simulink model "control_implementation"  (R2013b)
settings: Solver=ode45  StartTime=0.0  StopTime=10.0  RelTol=1e-3
libraries: simulink x1
settings Model: Creator=tvincent  LastModifiedBy=tvincent
settings DataIOCC: SignalLoggingSaveFormat=ModelDataLogs
settings DebuggingCC: UnderspecifiedInitializationDetection=Simplified  MultiTaskDSMMsg=warning  MultiTaskCondExecSysMsg=none  StrictBusMsg=None
settings RTWCC: IncludeERTFirstTime=on
settings GRTTargetCC: CodeReplacementLibrary=None  CPPClassGenCompliant=on

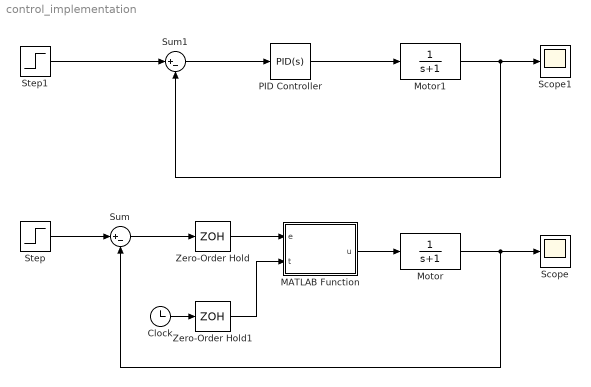
== system control_implementation ==
  Clock : Clock
  MATLAB Function : MATLAB Function  TreatAsAtomicUnit=on
  Motor : TransferFcn  Denominator=[1 1]
  Motor1 : TransferFcn  Denominator=[1 1]
  PID Controller : simulink/Continuous/PID Controller  Controller=PID  TimeDomain=Continuous-time  SampleTime=1  IntegratorMethod=Forward Euler  FilterMethod=Forward Euler  Form=Parallel  P=1  I=1  D=0  N=100  InitialConditionSource=internal  InitialConditionForIntegrator=0  InitialConditionForFilter=0  ExternalReset=none  LimitOutput=on  UpperSaturationLimit=10  LowerSaturationLimit=-10  LinearizeAsGain=on  AntiWindupMode=none  Kb=1  TrackingMode=off  Kt=1  PParamMin=[]  PParamMax=[]  IParamMin=[]  IParamMax=[]  DParamMin=[]  DParamMax=[]  NParamMin=[]  NParamMax=[]  KbParamMin=[]  KbParamMax=[]  KtParamMin=[]  KtParamMax=[]  POutMin=[]  POutMax=[]  IOutMin=[]  IOutMax=[]  DOutMin=[]  DOutMax=[]  NOutMin=[]  NOutMax=[]  KbOutMin=[]  KbOutMax=[]  KtOutMin=[]  KtOutMax=[]  IntegratorOutMin=[]  IntegratorOutMax=[]  FilterOutMin=[]  FilterOutMax=[]  SumOutMin=[]  SumOutMax=[]  SumI1OutMin=[]  SumI1OutMax=[]  SumI2OutMin=[]  SumI2OutMax=[]  SumI3OutMin=[]  SumI3OutMax=[]  SumDOutMin=[]  SumDOutMax=[]  SaturationOutMin=[]  SaturationOutMax=[]  IntegratorContinuousStateAttributes=''  IntegratorStateMustResolveToSignalObject=off  IntegratorRTWStateStorageClass=Auto  FilterContinuousStateAttributes=''  FilterStateMustResolveToSignalObject=off  FilterRTWStateStorageClass=Auto
  Scope : Scope
  Scope1 : Scope
  Step : Step  SampleTime=0
  Step1 : Step  SampleTime=0
  Sum : Sum  Inputs=|+-
  Sum1 : Sum  Inputs=|+-
  Zero-Order Hold : ZeroOrderHold  SampleTime=.001
  Zero-Order Hold1 : ZeroOrderHold  SampleTime=.001
  wires:
  Sum/1 -> Zero-Order Hold/1
  Zero-Order Hold/1 -> MATLAB Function/1(e)
  MATLAB Function/1(u) -> Motor/1
  Motor/1 -> Scope/1, Sum/2
  Step/1 -> Sum/1
  Sum1/1 -> PID Controller/1
  PID Controller/1 -> Motor1/1
  Motor1/1 -> Scope1/1, Sum1/2
  Step1/1 -> Sum1/1
  Clock/1 -> Zero-Order Hold1/1
  Zero-Order Hold1/1 -> MATLAB Function/2(t)

== matlab function control_implementation/MATLAB Function ==
  data: u output; e input; t input
function u = fcn(e,t)
%% Define Variables
% Control Gains
Kp=1;
Ki=1;
umax = 10;
% Memory variables
persistent I_past;
persistent t_past;
if isempty(I_past), I_past=0; end;
if isempty(t_past), t_past=0; end;

%% Calculate Controller
Ts = t - t_past;
% Integrator
I = I_past+e*Ts;
% PI control calculation
u = Kp*e+Ki*I;
if abs(u)>umax,
u = sign(u)*umax;
I = (u-Kp*e)/Ki;
end;
I_past=I;
t_past=t;
